simulink model "ModeSwitching"  (R2024a)
settings: Solver=FixedStepAuto  StartTime=0.0  StopTime=20  FixedStep=0.0005  RelTol=1e-3
values from neighbouring files (symbols this model uses):
  efficiency_map = efficiency_map / 100    [ModeSwitching_para.m]
  radius = 0.527    [ModeSwitching_para.m]
  s_thr = 0.2    [ModeSwitching_para.m]
  speed_rpm = [500,1000,1500,2000,2500,3000,3500,4000,4500,5000,5500,6000,6500,7000,7500,8000,8500,9000,9500,10000,10500,11000,11500,12000]    [ModeSwitching_para.m]
  torque_nm = [-600	-590	-580	-570	-560	-550	-540	-530	-520	-510	-500	-490	-480	-470	-460	-450	-440	-430	-420	-410	-400	-390	-380	-370	-360	-350	-340	-330	-320	-310	-300	-290	-280	-270	-260	-250	-240	-230	-220	-210	-200	-190	-180	-170	-160	-150	-140	-130	-120	-110	-100	-90	-80	-70	-60	-50	-40	-30	-20	-10	10	20	30	40	50	60	70	80	90	100	110	120	130	140	150	160	170	180	190	200	210	220	230	240	250	260	270	280	290	3 ...(+123 chars)    [ModeSwitching_para.m]
  v_min_s = 0.7    [ModeSwitching_para.m]
libraries: Solver_SF x1
(part 2 of 2)

== matlab function ModeSwitching/distribute Torque2 ==
  data: Torque input; T1 output; alpha_star input; T2 output; t input; alpha output
function [T1, T2, alpha] = fcn(Torque, alpha_star, t)
    dt = 0.1;
    t0 = 0.0;
    tEnd = (length(alpha_star)-1) * dt;   % 10.0 (若长度=101)

    % 1) 时间夹紧：避免超出范围
    if t <= t0
        alpha = alpha_star(1);
    elseif t >= tEnd
        alpha = alpha_star(end);
    else
        % 2) 线性插值（手写，便于 codegen，比 interp1 更稳）
        idx = floor((t - t0)/dt) + 1;     % idx in [1, length-1]
        if idx >= length(alpha_star)
            idx = length(alpha_star) - 1;
        end

        tL = t0 + (idx-1)*dt;
        w  = (t - tL)/dt;                 % 0~1
        alpha = (1-w)*alpha_star(idx) + w*alpha_star(idx+1);
    end
    T1 = alpha * Torque;
    T2 = (1-alpha) * Torque;
end

== matlab function ModeSwitching/MATLAB Function1 ==
  data: u input; k output
function k = torqueRatioNN(u)
% u 是一个2x1向量: [Treq; v_ms]
coder.extrinsic('evalin');

k = 0.0;                % 预设输出类型(标量double)
net = evalin('base','net');

u = u(:);               % 保证列向量
k = net(u);             % 直接推理：k = f(Treq, v)

% 限幅(如果你的k本来就是0~1)
if k < 0
    k = 0;
elseif k > 1
    k = 1;
end
end
